simulink model "manipulator2k20"  (Simulink 10.1)
settings: Solver=ode45  StartTime=0  StopTime=10  FixedStep=.01  RelTol=1e-3  EnableMultiTasking=on
values from neighbouring files (symbols this model uses):
  qic = Deval*q    [parsys.m]
settings Model: Creator=Janfron  LastModifiedBy=hrabi
settings DataIOCC: SignalLoggingSaveFormat=ModelDataLogs  SignalLoggingName=sigsOut
settings OptimizationCC: BooleanDataType=off  ExpressionDepthLimit=2147483647  InitFltsAndDblsToZero=on
settings DebuggingCC: SaveWithParameterizedLinksMsg=none  SignalResolutionControl=TryResolveAllWithWarning  MultiTaskDSMMsg=warning  MultiTaskCondExecSysMsg=none  FcnCallInpInsideContextMsg=warning  StateNameClashWarn=warning
settings HardwareCC: TargetUnknown=on
settings GRTTargetCC: TargetFcnLib=ansi_tfl_tmw.mat

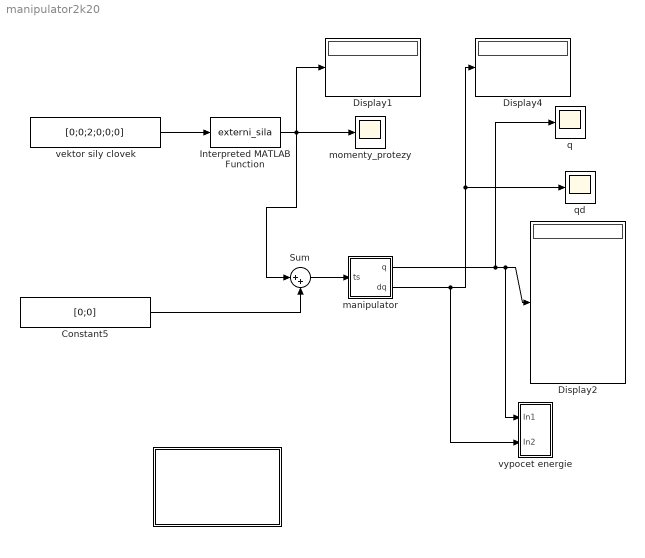
== system manipulator2k20 ==
  " " : Subsystem  mask{Parameter1=[]}
      mask prompts: Parameter1 "eval('parsys')"
      settings: OpenFcn=parsys
      mask Display: disp('parsys')
  Constant5 : Constant  Value=[0;0]
  Display1 : Display
  Display2 : Display
  Display4 : Display
  Interpreted MATLAB Function : MATLABFcn  MATLABFcn=externi_sila
  Sum : Sum  Inputs=|++
  manipulator : Subsystem
  momenty_protezy : Scope
  q : Scope
  qd : Scope
  vektor sily clovek : Constant  Value=[0;0;2;0;0;0]
  vypocet energie : Subsystem
  wires:
  manipulator/1(q) -> Display2/1, vypocet energie/1(In1), q/1
  manipulator/2(dq) -> Display4/1, qd/1, vypocet energie/2(In2)
  vektor sily clovek/1 -> Interpreted MATLAB Function/1
  Interpreted MATLAB Function/1 -> Sum/1, Display1/1, momenty_protezy/1
  Constant5/1 -> Sum/2
  Sum/1 -> manipulator/1(ts)

== system manipulator2k20/  ==

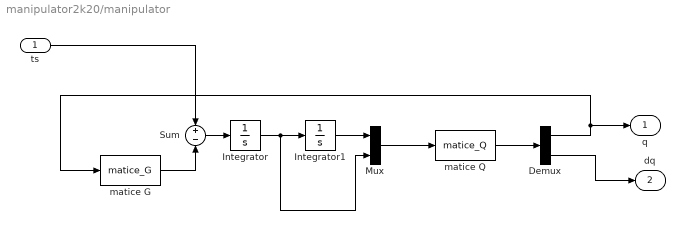
== system manipulator2k20/manipulator ==
  ts : Inport
  Demux : Demux  Outputs=[2 2]
      settings: DisplayOption=none
  Integrator : Integrator
  Integrator1 : Integrator  InitialCondition=qic
  Mux : Mux  Inputs=[2 2]
  Sum : Sum  Inputs=+-  InputSameDT=on  SaturateOnIntegerOverflow=on  OutDataTypeStr=Inherit: Same as first input
  matice G : MATLABFcn  MATLABFcn=matice_G
  matice Q : MATLABFcn  MATLABFcn=matice_Q
  q : Outport  VectorParamsAs1DForOutWhenUnconnected=off
  dq : Outport  Port=2  VectorParamsAs1DForOutWhenUnconnected=off
  wires:
  Integrator/1 -> Integrator1/1, Mux/2
  Mux/1 -> matice Q/1
  Sum/1 -> Integrator/1
  ts/1 -> Sum/1
  Demux/1 -> q/1, matice G/1
  Demux/2 -> dq/1
  matice G/1 -> Sum/2
  Integrator1/1 -> Mux/1
  matice Q/1 -> Demux/1

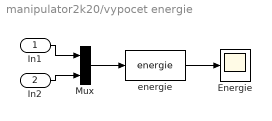
== system manipulator2k20/vypocet energie ==
  In1 : Inport
  In2 : Inport  Port=2
  Energie : Scope
  Mux : Mux  Inputs=[2 2]
  energie : MATLABFcn  MATLABFcn=energie  OutputDimensions=3
  wires:
  In2/1 -> Mux/2
  In1/1 -> Mux/1
  Mux/1 -> energie/1
  energie/1 -> Energie/1
